simulink model "power_PSS_example2"  (R2022a)
settings: Solver=ode23tb  StartTime=0.0  StopTime=25  MaxStep=1/60  RelTol=1e-3  EnableMultiTasking=on
InitFcn:
  | paraset
values from neighbouring files (symbols this model uses):
  delta = 0.1    [paraset.m]
  k = 0.01    [paraset.m]
  kappa = 1    [paraset.m]
undefined symbols (not defined in the file or in its folder): D1, Delta
libraries: spsGenericPowerSystemStabilizerLib x8, spsLoadFlowBusLib x6, spsThreePhaseParallelRLCLoadLib x4, spsThreePhasePISectionLineLib x4, spsSynchronousMachinepuStandardLib x4, spsExcitationSystemLib x4, spsMultiBandPowerSystemStabilizerLib x4, spsSteamTurbineandGovernorLib x4, spsThreePhaseTransformerTwoWindingsLib x4, spsDistributedParametersLineLib x3, spsThreePhaseBreakerLib x2, spsThreePhaseVIMeasurementLib x2
(part 1 of 2)
settings Model: FPTRunName=Active  ExtModeTrigMode=oneshot  ExtModeArmWhenConnect=off  Creator=The MathWorks, Inc.  LastModifiedBy=matsu
settings SolverCC: AlgebraicLoopSolver=TrustRegion
settings DataIOCC: SaveFormat=Array  SaveOutput=off  SaveTime=off  ReturnWorkspaceOutputs=off  TimeSaveName=t  SignalLoggingName=sigsOut
settings OptimizationCC: BlockReduction=off  BooleanDataType=off  ExpressionDepthLimit=2147483647  InitFltsAndDblsToZero=on  LifeSpan=inf
settings DebuggingCC: UnderspecifiedInitializationDetection=Classic  MergeDetectMultiDrivingBlocksExec=none  SignalResolutionControl=TryResolveAllWithWarning  MultiTaskDSMMsg=warning  MultiTaskCondExecSysMsg=none  FcnCallInpInsideContextMsg=warning  UnconnectedInputMsg=warning  UnconnectedLineMsg=warning  StateNameClashWarn=warning  SFUnexpectedBacktrackingDiag=warning  SFNoUnconditionalDefaultTransitionDiag=warning  SFExecutionAtInitializationDiag=none  SFMachineParentedDataDiag=warning  ArithmeticOperatorsInVariantConditions=warning
settings HardwareCC: ProdBitPerPointer=32  ProdBitPerSizeT=32  ProdBitPerPtrDiffT=32  ProdLargestAtomicFloat=None  ProdIntDivRoundTo=Undefined  ProdEndianess=Unspecified  ProdWordSize=32  ProdHWDeviceType=32-bit Generic  TargetUnknown=on
settings ModelReferenceCC: PropagateSignalLabelsOutOfModel=off
settings SFSimCC: SimUseLocalCustomCode=off  CustomCodeUndefinedFunction=UseInterfaceOnly
settings RTWCC: RTWUseLocalCustomCode=off
settings CodeAppCC: StateflowObjectComments=on
settings GRTTargetCC: TargetLangStandard=C89/C90 (ANSI)  CombineOutputUpdateFcns=off  GRTInterface=on
settings ConfigComp: CovMetricSettings=dw  CovSaveCumulativeToWorkspaceVar=on  CovSaveSingleToWorkspaceVar=on  CovExternalEMLEnable=off  CovSFcnEnable=off
settings SimscapeCC: SimscapeNormalizeSystem=off

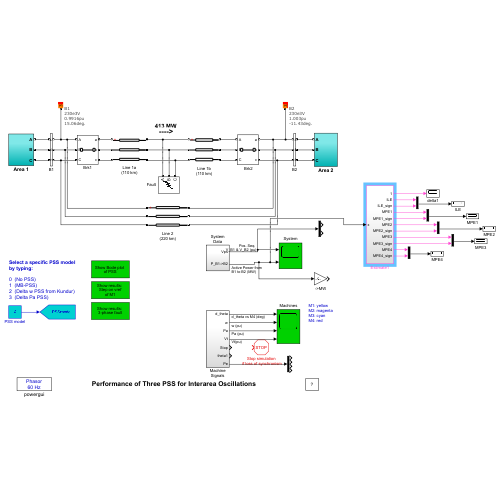
[thumbnail: Simulink's stored preview of the top-level diagram]
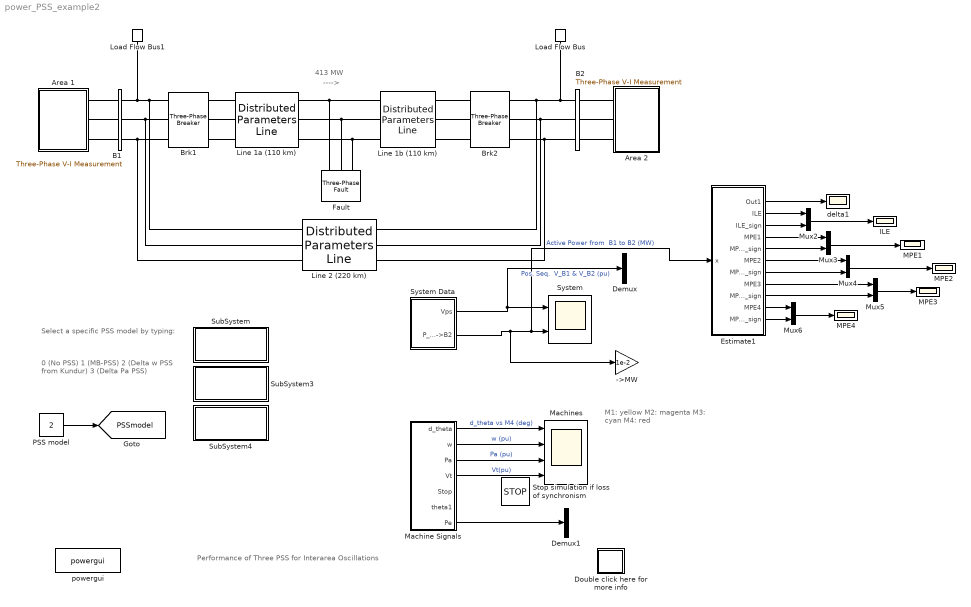
== system power_PSS_example2 ==
  note: Performance of Three PSS for Interarea Oscillations
  note: M1: yellow
      | M2: magenta
      | M3: cyan
      | M4: red
  note: ---->
  note: 413 MW
  note: Select a specific PSS model
      | by typing:
  note: 0  (No PSS)
      | 1  (MB-PSS)
      | 2  (Delta w PSS from Kundur)
      | 3  (Delta Pa PSS)
  " Brk2" : spsThreePhaseBreakerLib/Three-Phase Breaker  InitialState=closed  SwitchA=on  SwitchB=on  SwitchC=on  SwitchTimes=[1+6/60]  External=off  BreakerResistance=0.001  SnubberResistance=1e6  SnubberCapacitance=0  Measurements=None
      settings: AttributesFormatString=\n
  ->MW : Gain  Gain=1e-2  SaturateOnIntegerOverflow=on  OutDataTypeStr=Inherit: Same as input  ParamDataTypeStr=Inherit: Same as input
  Area 1 : Subsystem
  Area 2 : Subsystem
  B1 : spsThreePhaseVIMeasurementLib/Three-Phase V-I Measurement  VoltageMeasurement=phase-to-ground  SetLabelV=on  LabelV=Vabc_B1  Vpu=off  VpuLL=off  CurrentMeasurement=yes  SetLabelI=on  LabelI=Iabc_B1  Ipu=off  Pbase=100e6  Vbase=500e3  OutputType=Complex  PhasorSimulation=on  PSBequivalent=0
  B2 : spsThreePhaseVIMeasurementLib/Three-Phase V-I Measurement  VoltageMeasurement=phase-to-ground  SetLabelV=on  LabelV=Vabc_B2  Vpu=off  VpuLL=off  CurrentMeasurement=yes  SetLabelI=on  LabelI=Iabc_B2  Ipu=off  Pbase=100e6  Vbase=500e3  OutputType=Complex  PhasorSimulation=on  PSBequivalent=0
  Brk1 : spsThreePhaseBreakerLib/Three-Phase Breaker  InitialState=closed  SwitchA=on  SwitchB=on  SwitchC=on  SwitchTimes=[1+6/60]  External=off  BreakerResistance=0.001  SnubberResistance=inf  SnubberCapacitance=0  Measurements=None
      settings: AttributesFormatString=\n
  Demux : Demux  Outputs=2
  Demux1 : Demux
  Double click here for more info : Subsystem
      settings: OpenFcn=showdemo(bdroot(gcb))
      mask Display: disp('?')
  Estimate1 : Subsystem
  Fault : spsThreePhaseFaultLib/Three-Phase Fault  InitialStates=0  FaultA=on  FaultB=on  FaultC=on  GroundFault=on  SwitchTimes=[ 1 1+12/60]  External=off  SwitchStatus=NaN  FaultResistance=0.001  GroundResistance=0.001  SnubberResistance=inf  SnubberCapacitance=0  Measurements=None
  ILE : Scope
  Line 1a (110 km) : spsDistributedParametersLineLib/Distributed Parameters Line  Phases=3  Length=110  Frequency=60  Resistance=[0.0001*529 1.61]  Inductance=[0.001*529/(377) 0.0061]  Capacitance=[0.00175/529/(377) 5.2489e-9]  x1=[2.32637796386765e-08 228065.253428989 228064.749078735;376.991118430775 376.991118430775 376.991118430775;-1.32137751305166 0.640983254504953 -0.929809730908466]  x2=[1.11620897117682e-08 225636.373835133 225635.928060063;376.991118430775 376.991118430775 376.991118430775;-2.82766360003001 0.407410565435935 -1.16338269104508]  x3=[5.86477000241848e-11 336.016991920685 336.017366292842;376.991118430775 376.991118430775 376.991118430775;1.18739859871112 -2.54715832281008 2.16523641414879]  x4=[7.98351229776034e-11 1450.97195175507 1450.96987265642;376.991118430775 376.991118430775 376.991118430775;-1.93500873855342 0.484728016775275 -1.08606444535416]  x5=0.000622431770558027  V1=ones(3,3)  V2=ones(3,3)  I1=ones(3,3)  I2=ones(3,3)  nHarmo=1  Measurements=None  Decoupling=off  VsMag0=0  VrMag0=0  VsAngle0=0  VrAngle0=0  IsMag0=0  IrMag0=0  IsAngle0=0  IrAngle0=0
      settings: AttributesFormatString=\n  SourceProductBaseCode=PS
  Line 1b (110 km) : spsDistributedParametersLineLib/Distributed Parameters Line  Phases=3  Length=110  Frequency=60  Resistance=[0.0001*529 1.61]  Inductance=[0.001*529/(377) 0.0061]  Capacitance=[0.00175/529/(377) 5.2489e-9]  x1=[1.11620897117682e-08 225636.373835133 225635.928060063;376.991118430775 376.991118430775 376.991118430775;-2.82766360003001 0.407410565435935 -1.16338269104508]  x2=[3.02591716623452e-08 230641.661959582 230641.282002309;376.991118430775 376.991118430775 376.991118430775;2.60366923923542 0.178614649234263 -1.39217874313558]  x3=[7.01764132995704e-11 348.868575534709 348.868934214032;376.991118430775 376.991118430775 376.991118430775;1.39792395828996 -2.40713389014301 2.30526080396357]  x4=[6.82690946295777e-11 1438.06126547657 1438.05920047338;376.991118430775 376.991118430775 376.991118430775;-2.20731822356487 0.338658780991479 -1.23213368558469]  x5=0.000622431770558027  V1=ones(3,3)  V2=ones(3,3)  I1=ones(3,3)  I2=ones(3,3)  nHarmo=1  Measurements=None  Decoupling=off  VsMag0=0  VrMag0=0  VsAngle0=0  VrAngle0=0  IsMag0=0  IrMag0=0  IsAngle0=0  IrAngle0=0
      settings: AttributesFormatString=\n  SourceProductBaseCode=PS
  Line 2 (220 km) : spsDistributedParametersLineLib/Distributed Parameters Line  Phases=3  Length=220  Frequency=60  Resistance=[0.0001*529 1.61]  Inductance=[0.001*529/(377) 0.0061]  Capacitance=[0.00175/529/(377) 5.2489e-9]  x1=[1.24832194921319e-08 228066.159790877 228065.655439803;376.991118430775 376.991118430775 376.991118430775;-1.93381850732894 0.495470291490433 -1.0753226939196]  x2=[2.89327326949073e-08 230640.806586718 230640.426630747;376.991118430775 376.991118430775 376.991118430775;-1.98298217607113 0.0331007543902468 -1.53769263798565]  x3=[3.07384841100258e-11 335.618352779838 335.618719794473;376.991118430775 376.991118430775 376.991118430775;-2.78833319776652 -2.69313965469147 2.01925506825551]  x4=[1.71224684396664e-11 1425.65369023884 1425.6516439244;376.991118430775 376.991118430775 376.991118430775;-0.949321440854882 0.193205204918508 -1.37758726043151]  x5=0.00124486354111605  V1=ones(3,3)  V2=ones(3,3)  I1=ones(3,3)  I2=ones(3,3)  nHarmo=1  Measurements=None  Decoupling=off  VsMag0=0  VrMag0=0  VsAngle0=0  VrAngle0=0  IsMag0=0  IrMag0=0  IsAngle0=0  IrAngle0=0
      settings: AttributesFormatString=\n  SourceProductBaseCode=PS
  Load Flow Bus : spsLoadFlowBusLib/Load Flow Bus  LConnTagsString=a  Phases=single  Connectors=on one side  ID=B2  Vbase=230e3  Vref=1  Vangle=0  VLF=1.003  VLFb=1  VLFc=1  angleLF=-11.43  angleLFb=0  angleLFc=0
      settings: AttributesFormatString=%<ID>\n%<Vbase>V\n%<VLF>pu\n%<angleLF>deg.  SourceProductBaseCode=PS
  Load Flow Bus1 : spsLoadFlowBusLib/Load Flow Bus  LConnTagsString=a  Phases=single  Connectors=on one side  ID=B1  Vbase=230e3  Vref=1  Vangle=0  VLF=0.9916  VLFb=1  VLFc=1  angleLF=15.06  angleLFb=0  angleLFc=0
      settings: AttributesFormatString=%<ID>\n%<Vbase>V\n%<VLF>pu\n%<angleLF>deg.  SourceProductBaseCode=PS
  MPE{1..4} (4 alike) : Scope
  Machine Signals : Subsystem
  Machines : Scope  NumInputPorts=4
  Mux{2..6} (5 alike) : Mux  Inputs=2
  PSS model : Constant  Value=2
  Stop simulation if loss of synchronism : Stop
  SubSystem : Subsystem
      settings: OpenFcn=openfig('psbPSSbode.fig');
      mask Display: disp('Show Bode plot \nof PSS')
  SubSystem3 : Subsystem
      settings: OpenFcn=openfig('psbPSSstep.fig');
      mask Display: disp('Show results: \nStep on vref\nof M1')
  SubSystem4 : Subsystem
      settings: OpenFcn=openfig('psbPSSfault.fig');
      mask Display: disp('Show results: \n3-phase fault')
  System : Scope  NumInputPorts=2
  System Data : Subsystem
  delta1 : Scope
  powergui : spspowerguiLib/powergui  Priority=2  SimulationMode=Phasor  SampleTime=0  frequency=60  Iterations=50  frequencyindice=60  Pbase=100e6  ErrMax=0.0001  UnitsV=kV  UnitsW=MW  buscounter=0  FunctionMessages=off  echomessages=off  EnableUseOfTLC=off  CurrentSourceSwitches=off  DisableSnubberDevices=off  DisableRonSwitches=off  DisableVfSwitches=off  DisplayEquations=off  AutomaticDiscreteSolvers=off  SolverType=Tustin  Interpol=off  ExternalGateDelay=off  methode=off  Ts=0  x0status=blocks  SPID=off  SwTol=0  HookPort=off  NonlinearTolerance=1e-4  nMaxIteration=100  ContinueOnMaxIteration=off  RestoreLinks=warning  ResistiveCurrentMeasurement=off  Frange=logspace(0,3,50)  Ylog=off  Xlog=off  ShowGrid=off  save=off  variable=ZData  structure=0  ZoomFFT=on  StartTime=0.0  cycles=1  DisplayStyle=1  fundamental=60  FreqAxis=off  MaxFrequency=1000  frequencyindicesteady=1  RmsSteady=1  display=off
  tag scope: PSSmodel=global
  wires:
  Machine Signals/1(d_theta) -> Machines/1  "d_theta vs M4 (deg)"
  Machine Signals/2(w) -> Machines/2  "w (pu)"
  Machine Signals/3(Pa) -> Machines/3  "Pa (pu)"
  Machine Signals/4(Vt) -> Machines/4  "Vt(pu)"
  System Data/1(Vps) -> Demux/1, System/1  "Pos. Seq.  V_B1 & V_B2 (pu)"
  System Data/2(P_B1->B2) -> ->MW/1, Estimate1/1(x), System/2  "Active Power from  B1 to B2 (MW)"
  PSS model/1 -> [PSSmodel]
  Estimate1/4(MPE1) -> Mux3/1
  Estimate1/5(MPE1_sign) -> Mux3/2
  Estimate1/2(ILE) -> Mux2/1
  Mux2/1 -> ILE/1
  Mux5/1 -> MPE3/1
  Estimate1/9(MPE3_sign) -> Mux5/2
  Estimate1/8(MPE3) -> Mux5/1
  Mux6/1 -> MPE4/1
  Estimate1/11(MPE4_sign) -> Mux6/2
  Estimate1/7(MPE2_sign) -> Mux4/2
  Estimate1/1(Out1) -> delta1/1
  Estimate1/3(ILE_sign) -> Mux2/2
  Estimate1/6(MPE2) -> Mux4/1
  Mux4/1 -> MPE2/1
  Estimate1/10(MPE4) -> Mux6/1
  Mux3/1 -> MPE1/1
  Machine Signals/7(Pe) -> Demux1/1
  connections:
  Brk1/RConn1 -- Line 1a (110 km)/LConn1
  Brk1/RConn2 -- Line 1a (110 km)/LConn2
  Brk1/RConn3 -- Line 1a (110 km)/LConn3
  Line 1b (110 km)/LConn1 -- Line 1a (110 km)/RConn1 -- Fault/LConn1
  Line 1b (110 km)/LConn2 -- Line 1a (110 km)/RConn2 -- Fault/LConn2
  Line 1a (110 km)/RConn3 -- Line 1b (110 km)/LConn3 -- Fault/LConn3
  Line 1b (110 km)/RConn1 -- " Brk2"/LConn1
  Line 1b (110 km)/RConn2 -- " Brk2"/LConn2
  Line 1b (110 km)/RConn3 -- " Brk2"/LConn3
  Area 1/RConn2 -- B1/LConn2
  Area 1/RConn1 -- B1/LConn1
  Area 1/RConn3 -- B1/LConn3
  B1/RConn2 -- Brk1/LConn2 -- Line 2 (220 km)/LConn2
  B1/RConn1 -- Brk1/LConn1 -- Line 2 (220 km)/LConn1 -- Load Flow Bus1/LConn1
  B1/RConn3 -- Brk1/LConn3 -- Line 2 (220 km)/LConn3
  B2/RConn2 -- Area 2/LConn2
  B2/RConn1 -- Area 2/LConn1
  B2/RConn3 -- Area 2/LConn3
  B2/LConn2 -- " Brk2"/RConn2 -- Line 2 (220 km)/RConn2
  B2/LConn1 -- " Brk2"/RConn1 -- Line 2 (220 km)/RConn1 -- Load Flow Bus/LConn1
  B2/LConn3 -- " Brk2"/RConn3 -- Line 2 (220 km)/RConn3

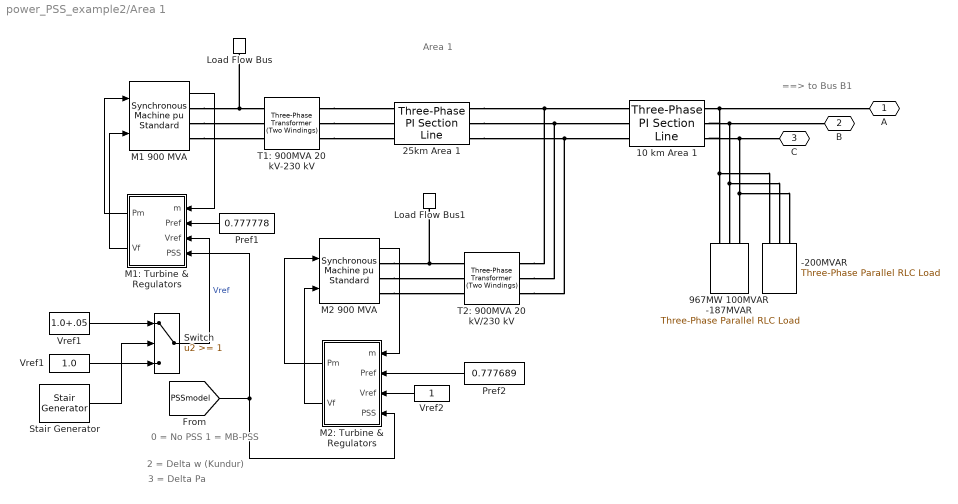
== system power_PSS_example2/Area 1 ==
  note: Area 1
  note: ==> to Bus B1
  note: 0 = No PSS
      | 1 = MB-PSS
  note: 3 = Delta Pa
  note: 2 = Delta w (Kundur)
  -200MVAR : spsThreePhaseParallelRLCLoadLib/Three-Phase Parallel RLC Load  LConnTagsString=A|B|C  Configuration=Y (grounded)  NominalVoltage=230e3  Vabc=[1e3 1e3 1e3]  Vabcp=[1e3 1e3 1e3]  NominalFrequency=60  UnbalancedPower=off  ActivePower=0  InductivePower=0  CapacitivePower=200e6  Pabc=[10e3 9e3 11e3]  QLabc=[100 90 110]  QCabc=[100 90 110]  Pabcp=[10e3 9e3 11e3]  QLabcp=[100 90 110]  QCabcp=[100 90 110]  Measurements=None  LoadType=constant Z
  10 km Area 1 : spsThreePhasePISectionLineLib/Three-Phase PI Section Line  LConnTagsString=a|b|c  RConnTagsString=A|B|C  Length=10  Frequency=60  Resistances=[0.0001*529 1.61]  Inductances=[0.001*529/(377) 0.0061]  Capacitances=[0.00175/529/(377) 5.2489e-9]
  25km Area 1 : spsThreePhasePISectionLineLib/Three-Phase PI Section Line  LConnTagsString=a|b|c  RConnTagsString=A|B|C  Length=25  Frequency=60  Resistances=[0.0001*529 1.61]  Inductances=[0.001*529/(377) 0.0061]  Capacitances=[0.00175/529/(377) 5.2489e-9]
  967MW 100MVAR -187MVAR : spsThreePhaseParallelRLCLoadLib/Three-Phase Parallel RLC Load  LConnTagsString=A|B|C  Configuration=Y (grounded)  NominalVoltage=230e3  Vabc=[1e3 1e3 1e3]  Vabcp=[1e3 1e3 1e3]  NominalFrequency=60  UnbalancedPower=off  ActivePower=967000000  InductivePower=100e6  CapacitivePower=187e6  Pabc=[10e3 9e3 11e3]  QLabc=[100 90 110]  QCabc=[100 90 110]  Pabcp=[10e3 9e3 11e3]  QLabcp=[100 90 110]  QCabcp=[100 90 110]  Measurements=None  LoadType=constant Z
  Load Flow Bus : spsLoadFlowBusLib/Load Flow Bus  LConnTagsString=a  Phases=single  Connectors=on one side  ID=M1_Area1  Vbase=20e3  Vref=1  Vangle=0  VLF=1  VLFb=1  VLFc=1  angleLF=10.22  angleLFb=0  angleLFc=0
      settings: AttributesFormatString=%<ID>\n%<Vbase>V\n%<VLF>pu\n%<angleLF>deg.  SourceProductBaseCode=PS
  Load Flow Bus1 : spsLoadFlowBusLib/Load Flow Bus  LConnTagsString=a  Phases=single  Connectors=on one side  ID=M2_Area1  Vbase=20e3  Vref=1  Vangle=0  VLF=1  VLFb=1  VLFc=1  angleLF=0  angleLFb=0  angleLFc=0
      settings: AttributesFormatString=%<ID>\n%<Vbase>V\n%<VLF>pu\n%<angleLF>deg.  SourceProductBaseCode=PS
  M1 900 MVA : spsSynchronousMachinepuStandardLib/Synchronous Machine pu Standard  PresetModel=No  MechanicalLoad=Mechanical power Pm  ShowDetailedParameters=on  RotorType=Round  Units=per unit standard parameters  MeasurementBus=off  NominalParameters="[900E6  20000   60 ]"  Reactances1=[1.8 .3 .25 1.7 .55 .25 .2]  Reactances2=[ 1.305, 0.296, 0.252, 0.474, 0.243, 0.18 ]  dAxisTimeConstants=Open-circuit  qAxisTimeConstants=Open-circuit  TimeConstants1=[]  TimeConstants2=[8 .03 .4 .05]  TimeConstants3=[]  TimeConstants4=[]  TimeConstants5=[ 1.01, 0.053, 0.1 ]  TimeConstants6=[]  TimeConstants7=[]  TimeConstants8=[]  StatorResistance=0.0025  Mechanical=[ 6.5 0 4]  PolePairs=4  InitialConditions=[0 -31.4247 0.784453 0.784453 0.784453 2.7401 -117.26 122.74 1.83395]  SetSaturation=off  Saturation=[0.6404,0.7127,0.8441,0.9214,0.9956,1.082,1.19,1.316,1.457;0.7,0.7698,0.8872,0.9466,0.9969,1.046,1.1,1.151,1.201]  LoadFlowParameters=[1 700000000 0 0 0]  TsPowergui=0  TsBlock=-1  IterativeModel=Trapezoidal non iterative  IterativeDiscreteModel=Trapezoidal non iterative  BusType=PV  Pref=700000000  Qref=0  Qmin=-Inf  Qmax=Inf  PLF=0  QLF=0
      settings: SourceProductBaseCode=PS
  M1: Turbine & Regulators : Subsystem
  M2 900 MVA : spsSynchronousMachinepuStandardLib/Synchronous Machine pu Standard  PresetModel=No  MechanicalLoad=Mechanical power Pm  ShowDetailedParameters=on  RotorType=Round  Units=per unit standard parameters  MeasurementBus=off  NominalParameters="[900E6  20000   60 ]"  Reactances1=[1.8 .3 .25 1.7 .55 .25 .2]  Reactances2=[ 1.305, 0.296, 0.252, 0.474, 0.243, 0.18 ]  dAxisTimeConstants=Open-circuit  qAxisTimeConstants=Open-circuit  TimeConstants1=[]  TimeConstants2=[8 .03 .4 .05]  TimeConstants3=[]  TimeConstants4=[]  TimeConstants5=[ 1.01, 0.053, 0.1 ]  TimeConstants6=[]  TimeConstants7=[]  TimeConstants8=[]  StatorResistance=0.0025  Mechanical=[ 6.5 0 4]  PolePairs=4  InitialConditions=[0 -42.8075 0.788608 0.788608 0.788608 -9.54571 -129.546 110.454 1.86756]  SetSaturation=off  Saturation=[0.6404,0.7127,0.8441,0.9214,0.9956,1.082,1.19,1.316,1.457;0.7,0.7698,0.8872,0.9466,0.9969,1.046,1.1,1.151,1.201]  LoadFlowParameters=[2 700000000 0 0 0]  TsPowergui=0  TsBlock=-1  IterativeModel=Trapezoidal non iterative  IterativeDiscreteModel=Trapezoidal non iterative  BusType=swing  Pref=0  Qref=0  Qmin=-Inf  Qmax=Inf  PLF=0  QLF=0
      settings: SourceProductBaseCode=PS
  M2: Turbine & Regulators : Subsystem
  Pref1 : Constant  Value=0.777778
  Pref2 : Constant  Value=0.777689
  Stair Generator : spsStairGeneratorLib/Stair Generator  t=[0 1 1.2]*100  e=[0 1 0 ]  Ts=0
  Switch : Switch  Threshold=1  SaturateOnIntegerOverflow=off
  T1: 900MVA 20 kV-230 kV : spsThreePhaseTransformerTwoWindingsLib/Three-Phase Transformer (Two Windings)  Winding1Connection=Delta (D1)  Winding2Connection=Yg  CoreType=Three single-phase transformers  SetSaturation=off  Hysteresis=off  DataFile='hysteresis'  SetInitialFlux=off  Measurements=None  UNITS=pu  NominalPower="[ 900e6   60 ]"  Winding1="[ 20e3  1e-6   0  ]"  Winding2="[ 230e3  1e-6   0.15 ]"  Rm=500  Lm=500  L0=0.5  Saturation="[ 0,0  ;  0.005,1.2  ;  1.0,1.4 ]"  InitialFluxes=[ 0.8 , -0.8 , 0.7 ]  BreakLoop=off  DiscreteSolver=Trapezoidal iterative  DataType=off  TransfoNumber=0
  T2: 900MVA 20 kV/230 kV : spsThreePhaseTransformerTwoWindingsLib/Three-Phase Transformer (Two Windings)  Winding1Connection=Delta (D1)  Winding2Connection=Yg  CoreType=Three single-phase transformers  SetSaturation=off  Hysteresis=off  DataFile='hysteresis'  SetInitialFlux=off  Measurements=None  UNITS=pu  NominalPower=[ 900e6 60 ]  Winding1="[ 20e3 1e-6  0.0]"  Winding2=[ 230e3 1e-6 0.15]  Rm=500  Lm=500  L0=0.5  Saturation="[ 0,0  ;  0.005,1.2  ;  1.0,1.4 ]"  InitialFluxes=[ 0.8 , -0.8 , 0.7 ]  BreakLoop=off  DiscreteSolver=Trapezoidal iterative  DataType=off  TransfoNumber=0
  Vref1 : Constant  Value=1.0
  "Vref1 " : Constant  Value=1.0+.05
  Vref2 : Constant
  " A" : PMIOPort  Side=Right
  " B" : PMIOPort  Port=2  Side=Right
  " C" : PMIOPort  Port=3  Side=Right
  wires:
  Pref1/1 -> M1: Turbine & Regulators/2(Pref)
  Switch/1 -> M1: Turbine & Regulators/3(Vref)  "Vref"
  Stair Generator/1 -> Switch/2
  [PSSmodel] -> M1: Turbine & Regulators/4(PSS), M2: Turbine & Regulators/4(PSS)
  Pref2/1 -> M2: Turbine & Regulators/2(Pref)
  Vref2/1 -> M2: Turbine & Regulators/3(Vref)
  Vref1/1 -> Switch/3
  "Vref1 "/1 -> Switch/1
  M2 900 MVA/1 -> M2: Turbine & Regulators/1(m)
  M2: Turbine & Regulators/1(Pm) -> M2 900 MVA/1
  M2: Turbine & Regulators/2(Vf) -> M2 900 MVA/2
  M1: Turbine & Regulators/1(Pm) -> M1 900 MVA/1
  M1: Turbine & Regulators/2(Vf) -> M1 900 MVA/2
  M1 900 MVA/1 -> M1: Turbine & Regulators/1(m)
  connections:
  T1: 900MVA 20 kV-230 kV/RConn1 -- 25km Area 1/LConn1
  T1: 900MVA 20 kV-230 kV/RConn2 -- 25km Area 1/LConn2
  M2 900 MVA/RConn1 -- T2: 900MVA 20 kV/230 kV/LConn1 -- Load Flow Bus1/LConn1
  M2 900 MVA/RConn2 -- T2: 900MVA 20 kV/230 kV/LConn2
  M2 900 MVA/RConn3 -- T2: 900MVA 20 kV/230 kV/LConn3
  T1: 900MVA 20 kV-230 kV/RConn3 -- 25km Area 1/LConn3
  10 km Area 1/RConn1 -- " A"/RConn1 -- 967MW 100MVAR -187MVAR/LConn1 -- -200MVAR/LConn1
  10 km Area 1/RConn2 -- " B"/RConn1 -- 967MW 100MVAR -187MVAR/LConn2 -- -200MVAR/LConn2
  10 km Area 1/RConn3 -- " C"/RConn1 -- 967MW 100MVAR -187MVAR/LConn3 -- -200MVAR/LConn3
  M1 900 MVA/RConn1 -- T1: 900MVA 20 kV-230 kV/LConn1 -- Load Flow Bus/LConn1
  M1 900 MVA/RConn2 -- T1: 900MVA 20 kV-230 kV/LConn2
  M1 900 MVA/RConn3 -- T1: 900MVA 20 kV-230 kV/LConn3
  25km Area 1/RConn2 -- 10 km Area 1/LConn2 -- T2: 900MVA 20 kV/230 kV/RConn2
  25km Area 1/RConn1 -- 10 km Area 1/LConn1 -- T2: 900MVA 20 kV/230 kV/RConn1
  25km Area 1/RConn3 -- 10 km Area 1/LConn3 -- T2: 900MVA 20 kV/230 kV/RConn3

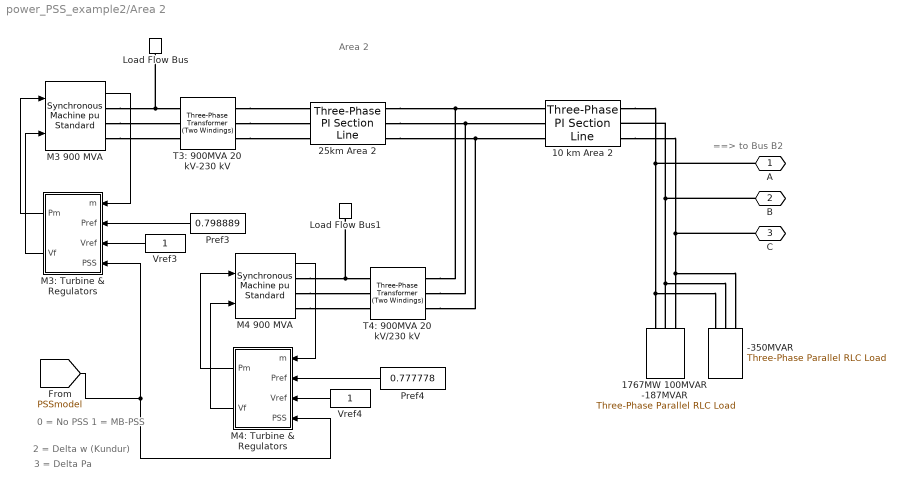
== system power_PSS_example2/Area 2 ==
  note: 2 = Delta w (Kundur)
  note: 3 = Delta Pa
  note: 0 = No PSS
      | 1 = MB-PSS
  note: ==> to Bus B2
  note: Area 2
  -350MVAR : spsThreePhaseParallelRLCLoadLib/Three-Phase Parallel RLC Load  LConnTagsString=A|B|C  Configuration=Y (grounded)  NominalVoltage=230e3  Vabc=[1e3 1e3 1e3]  Vabcp=[1e3 1e3 1e3]  NominalFrequency=60  UnbalancedPower=off  ActivePower=0  InductivePower=0  CapacitivePower=350e6  Pabc=[10e3 9e3 11e3]  QLabc=[100 90 110]  QCabc=[100 90 110]  Pabcp=[10e3 9e3 11e3]  QLabcp=[100 90 110]  QCabcp=[100 90 110]  Measurements=None  LoadType=constant Z
  10 km Area 2 : spsThreePhasePISectionLineLib/Three-Phase PI Section Line  LConnTagsString=a|b|c  RConnTagsString=A|B|C  Length=10  Frequency=60  Resistances=[0.0001*529 1.61]  Inductances=[0.001*529/(377) 0.0061]  Capacitances=[0.00175/529/(377) 5.2489e-9]
  1767MW 100MVAR -187MVAR : spsThreePhaseParallelRLCLoadLib/Three-Phase Parallel RLC Load  LConnTagsString=A|B|C  Configuration=Y (grounded)  NominalVoltage=230e3  Vabc=[1e3 1e3 1e3]  Vabcp=[1e3 1e3 1e3]  NominalFrequency=60  UnbalancedPower=off  ActivePower=1767000000  InductivePower=100e6  CapacitivePower=187e6  Pabc=[10e3 9e3 11e3]  QLabc=[100 90 110]  QCabc=[100 90 110]  Pabcp=[10e3 9e3 11e3]  QLabcp=[100 90 110]  QCabcp=[100 90 110]  Measurements=None  LoadType=constant Z
  25km Area 2 : spsThreePhasePISectionLineLib/Three-Phase PI Section Line  LConnTagsString=a|b|c  RConnTagsString=A|B|C  Length=25  Frequency=60  Resistances=[0.0001*529 1.61]  Inductances=[0.001*529/(377) 0.0061]  Capacitances=[0.00175/529/(377) 5.2489e-9]
  Load Flow Bus : spsLoadFlowBusLib/Load Flow Bus  LConnTagsString=a  Phases=single  Connectors=on one side  ID=M3_Area2  Vbase=20e3  Vref=1  Vangle=0  VLF=1  VLFb=1  VLFc=1  angleLF=-15.88  angleLFb=0  angleLFc=0
      settings: AttributesFormatString=%<ID>\n%<Vbase>V\n%<VLF>pu\n%<angleLF>deg.  SourceProductBaseCode=PS
  Load Flow Bus1 : spsLoadFlowBusLib/Load Flow Bus  LConnTagsString=a  Phases=single  Connectors=on one side  ID=M4_Area2  Vbase=20e3  Vref=1  Vangle=0  VLF=1  VLFb=1  VLFc=1  angleLF=-26.53  angleLFb=0  angleLFc=0
      settings: AttributesFormatString=%<ID>\n%<Vbase>V\n%<VLF>pu\n%<angleLF>deg.  SourceProductBaseCode=PS
  M3 900 MVA : spsSynchronousMachinepuStandardLib/Synchronous Machine pu Standard  PresetModel=No  MechanicalLoad=Mechanical power Pm  ShowDetailedParameters=on  RotorType=Round  Units=per unit standard parameters  MeasurementBus=off  NominalParameters="[900E6  20000   60 ]"  Reactances1=[1.8 .3 .25 1.7 .55 .25 .2]  Reactances2=[ 1.305, 0.296, 0.252, 0.474, 0.243, 0.18 ]  dAxisTimeConstants=Open-circuit  qAxisTimeConstants=Open-circuit  TimeConstants1=[]  TimeConstants2=[8 .03 .4 .05]  TimeConstants3=[]  TimeConstants4=[]  TimeConstants5=[ 1.01, 0.053, 0.1 ]  TimeConstants6=[]  TimeConstants7=[]  TimeConstants8=[]  StatorResistance=0.0025  Mechanical=[ 6.175 0 4]  PolePairs=4  InitialConditions=[0 -56.3243 0.8041 0.8041 0.8041 -22.4087 -142.409 97.5913 1.85092]  SetSaturation=off  Saturation=[0.6404,0.7127,0.8441,0.9214,0.9956,1.082,1.19,1.316,1.457;0.7,0.7698,0.8872,0.9466,0.9969,1.046,1.1,1.151,1.201]  LoadFlowParameters=[1 719000000 0 0 0]  TsPowergui=0  TsBlock=-1  IterativeModel=Trapezoidal non iterative  IterativeDiscreteModel=Trapezoidal non iterative  BusType=PV  Pref=719000000  Qref=0  Qmin=-Inf  Qmax=Inf  PLF=0  QLF=0
      settings: SourceProductBaseCode=PS
  M3: Turbine & Regulators : Subsystem
  M4 900 MVA : spsSynchronousMachinepuStandardLib/Synchronous Machine pu Standard  PresetModel=No  MechanicalLoad=Mechanical power Pm  ShowDetailedParameters=on  RotorType=Round  Units=per unit standard parameters  MeasurementBus=off  NominalParameters="[900E6  20000   60 ]"  Reactances1=[1.8 .3 .25 1.7 .55 .25 .2]  Reactances2=[ 1.305, 0.296, 0.252, 0.474, 0.243, 0.18 ]  dAxisTimeConstants=Open-circuit  qAxisTimeConstants=Open-circuit  TimeConstants1=[]  TimeConstants2=[8 .03 .4 .05]  TimeConstants3=[]  TimeConstants4=[]  TimeConstants5=[ 1.01, 0.053, 0.1 ]  TimeConstants6=[]  TimeConstants7=[]  TimeConstants8=[]  StatorResistance=0.0025  Mechanical=[ 6.175 0 4]  PolePairs=4  InitialConditions=[0 -67.7513 0.783185 0.783185 0.783185 -33.268 -153.268 86.732 1.82209]  SetSaturation=off  Saturation=[0.6404,0.7127,0.8441,0.9214,0.9956,1.082,1.19,1.316,1.457;0.7,0.7698,0.8872,0.9466,0.9969,1.046,1.1,1.151,1.201]  LoadFlowParameters=[1 700000000 0 0 0]  TsPowergui=0  TsBlock=-1  IterativeModel=Trapezoidal non iterative  IterativeDiscreteModel=Trapezoidal non iterative  BusType=PV  Pref=700000000  Qref=0  Qmin=-Inf  Qmax=Inf  PLF=0  QLF=0
      settings: SourceProductBaseCode=PS
  M4: Turbine & Regulators : Subsystem
  Pref3 : Constant  Value=0.798889
  Pref4 : Constant  Value=0.777778
  T3: 900MVA 20 kV-230 kV : spsThreePhaseTransformerTwoWindingsLib/Three-Phase Transformer (Two Windings)  Winding1Connection=Delta (D1)  Winding2Connection=Yg  CoreType=Three single-phase transformers  SetSaturation=off  Hysteresis=off  DataFile='hysteresis'  SetInitialFlux=off  Measurements=None  UNITS=pu  NominalPower="[ 900e6   60 ]"  Winding1="[ 20e3  1e-6   0  ]"  Winding2="[ 230e3  1e-6   0.15 ]"  Rm=500  Lm=500  L0=0.5  Saturation="[ 0,0  ;  0.005,1.2  ;  1.0,1.4 ]"  InitialFluxes=[ 0.8 , -0.8 , 0.7 ]  BreakLoop=off  DiscreteSolver=Trapezoidal iterative  DataType=off  TransfoNumber=0
  T4: 900MVA 20 kV/230 kV : spsThreePhaseTransformerTwoWindingsLib/Three-Phase Transformer (Two Windings)  Winding1Connection=Delta (D1)  Winding2Connection=Yg  CoreType=Three single-phase transformers  SetSaturation=off  Hysteresis=off  DataFile='hysteresis'  SetInitialFlux=off  Measurements=None  UNITS=pu  NominalPower=[ 900e6 60 ]  Winding1="[ 20e3 1e-6  0.0]"  Winding2=[ 230e3 1e-6 0.15]  Rm=500  Lm=500  L0=0.5  Saturation="[ 0,0  ;  0.005,1.2  ;  1.0,1.4 ]"  InitialFluxes=[ 0.8 , -0.8 , 0.7 ]  BreakLoop=off  DiscreteSolver=Trapezoidal iterative  DataType=off  TransfoNumber=0
  Vref3 : Constant
  Vref4 : Constant
  A : PMIOPort  Side=Left
  B : PMIOPort  Port=2  Side=Left
  C : PMIOPort  Port=3  Side=Left
  wires:
  [PSSmodel] -> M3: Turbine & Regulators/4(PSS), M4: Turbine & Regulators/4(PSS)
  Pref3/1 -> M3: Turbine & Regulators/2(Pref)
  Vref3/1 -> M3: Turbine & Regulators/3(Vref)
  Pref4/1 -> M4: Turbine & Regulators/2(Pref)
  Vref4/1 -> M4: Turbine & Regulators/3(Vref)
  M3 900 MVA/1 -> M3: Turbine & Regulators/1(m)
  M3: Turbine & Regulators/2(Vf) -> M3 900 MVA/2
  M3: Turbine & Regulators/1(Pm) -> M3 900 MVA/1
  M4: Turbine & Regulators/1(Pm) -> M4 900 MVA/1
  M4: Turbine & Regulators/2(Vf) -> M4 900 MVA/2
  M4 900 MVA/1 -> M4: Turbine & Regulators/1(m)
  connections:
  M3 900 MVA/RConn3 -- T3: 900MVA 20 kV-230 kV/LConn3
  M3 900 MVA/RConn2 -- T3: 900MVA 20 kV-230 kV/LConn2
  M3 900 MVA/RConn1 -- T3: 900MVA 20 kV-230 kV/LConn1 -- Load Flow Bus/LConn1
  T3: 900MVA 20 kV-230 kV/RConn3 -- 25km Area 2/LConn3
  M4 900 MVA/RConn3 -- T4: 900MVA 20 kV/230 kV/LConn3
  M4 900 MVA/RConn2 -- T4: 900MVA 20 kV/230 kV/LConn2
  M4 900 MVA/RConn1 -- T4: 900MVA 20 kV/230 kV/LConn1 -- Load Flow Bus1/LConn1
  T3: 900MVA 20 kV-230 kV/RConn2 -- 25km Area 2/LConn2
  T3: 900MVA 20 kV-230 kV/RConn1 -- 25km Area 2/LConn1
  25km Area 2/RConn2 -- 10 km Area 2/LConn2 -- T4: 900MVA 20 kV/230 kV/RConn2
  25km Area 2/RConn1 -- 10 km Area 2/LConn1 -- T4: 900MVA 20 kV/230 kV/RConn1
  25km Area 2/RConn3 -- 10 km Area 2/LConn3 -- T4: 900MVA 20 kV/230 kV/RConn3
  10 km Area 2/RConn1 -- 1767MW 100MVAR -187MVAR/LConn1 -- -350MVAR/LConn1 -- A/RConn1
  1767MW 100MVAR -187MVAR/LConn2 -- -350MVAR/LConn2 -- 10 km Area 2/RConn2 -- B/RConn1
  10 km Area 2/RConn3 -- 1767MW 100MVAR -187MVAR/LConn3 -- -350MVAR/LConn3 -- C/RConn1

== system power_PSS_example2/Double click here for more info ==

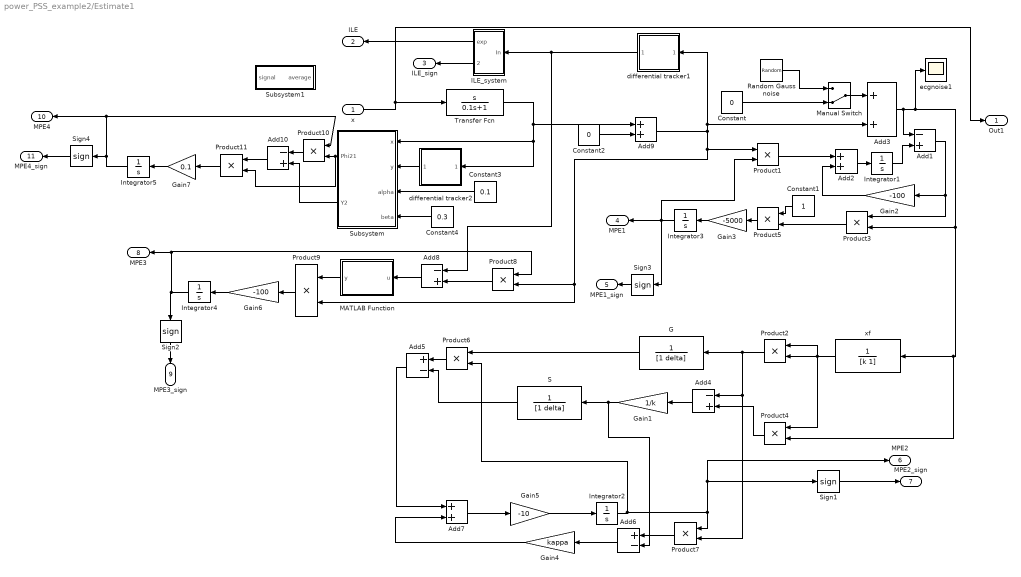
== system power_PSS_example2/Estimate1 ==
  x : Inport
  Add{1,4,8,10} (4 alike) : Sum  Inputs=-+
  Add{2..3,7,9} (4 alike) : Sum
  Add5 : Sum  Inputs=+-
  Add6 : Sum  Inputs=+-
  Constant : Constant  Value=0
  Constant1 : Constant
  Constant2 : Constant  Value=0
  Constant3 : Constant  Value=0.1
  Constant4 : Constant  Value=0.3
  G : TransferFcn  Denominator=[1 delta]
  Gain1 : Gain  Gain=1/k
  Gain2 : Gain  Gain=-100
  Gain3 : Gain  Gain=-5000
  Gain4 : Gain  Gain=kappa
  Gain5 : Gain  Gain=-10
  Gain6 : Gain  Gain=-100
  Gain7 : Gain  Gain=0.1
  ILE_system : Subsystem
  Integrator{1..5} (5 alike) : Integrator
  MATLAB Function : MATLAB Function  TreatAsAtomicUnit=on
  Manual Switch : ManualSwitch  CurrentSetting=0
  Product{1..11} (11 alike) : Product  RndMeth=Zero
  Random Gauss noise : RandomNumber  Variance=0.0001  SampleTime=0
  S : TransferFcn  Denominator=[1 delta]
  Sign{1..4} (4 alike) : Signum
  Subsystem : Subsystem
  Subsystem1 : Subsystem
  Transfer Fcn : TransferFcn  Numerator=[1 0]  Denominator=[0.1 1]
  differential tracker1 : Subsystem
  differential tracker2 : Subsystem
  ecgnoise1 : Scope
  xf : TransferFcn  Denominator=[k 1]
  Out1 : Outport  VectorParamsAs1DForOutWhenUnconnected=off
  ILE : Outport  Port=2  VectorParamsAs1DForOutWhenUnconnected=off
  ILE_sign : Outport  Port=3  VectorParamsAs1DForOutWhenUnconnected=off
  MPE1 : Outport  Port=4  VectorParamsAs1DForOutWhenUnconnected=off
  MPE1_sign : Outport  Port=5  VectorParamsAs1DForOutWhenUnconnected=off
  MPE2 : Outport  Port=6  VectorParamsAs1DForOutWhenUnconnected=off
  MPE2_sign : Outport  Port=7  VectorParamsAs1DForOutWhenUnconnected=off
  MPE3 : Outport  Port=8  VectorParamsAs1DForOutWhenUnconnected=off
  MPE3_sign : Outport  Port=9  VectorParamsAs1DForOutWhenUnconnected=off
  MPE4 : Outport  Port=10  VectorParamsAs1DForOutWhenUnconnected=off
  MPE4_sign : Outport  Port=11  VectorParamsAs1DForOutWhenUnconnected=off
  wires:
  Integrator1/1 -> Add1/2
  Add3/1 -> Product4/2, xf/1, Product3/2, ecgnoise1/1, Add1/1
  Manual Switch/1 -> Add3/1
  Random Gauss noise/1 -> Manual Switch/1
  Constant/1 -> Manual Switch/2
  Product1/1 -> Add2/1
  Gain3/1 -> Integrator3/1
  Add1/1 -> Product3/1, Gain2/1
  Product5/1 -> Gain3/1
  Gain2/1 -> Add2/2
  Add2/1 -> Integrator1/1
  Product3/1 -> Product5/2
  Constant1/1 -> Product5/1
  Integrator3/1 -> Sign3/1, MPE1/1, Product1/2
  ILE_system/2(sign) -> ILE_sign/1
  ILE_system/1(exp) -> ILE/1
  differential tracker1/1(diff_estimate) -> Add8/1, ILE_system/1(In)
  xf/1 -> Product4/1, Product2/1, Product2/2
  Product2/1 -> Product7/2, Add4/1, G/1
  Product4/1 -> Add4/2
  Add4/1 -> Gain1/1
  Gain1/1 -> Add6/2, S/1
  G/1 -> Product6/1
  Integrator2/1 -> Sign1/1, MPE2/1, Product7/1, Product6/2
  Product6/1 -> Add5/1
  S/1 -> Add5/2
  Product7/1 -> Add6/1
  Add6/1 -> Gain4/1
  Add5/1 -> Add7/1
  Gain4/1 -> Add7/2
  Add7/1 -> Gain5/1
  Gain5/1 -> Integrator2/1
  Sign1/1 -> MPE2_sign/1
  Product8/1 -> Add8/2
  Add8/1 -> MATLAB Function/1(u)
  MATLAB Function/1(y) -> Product9/1
  Product9/1 -> Gain6/1
  Gain6/1 -> Integrator4/1
  Integrator4/1 -> Sign2/1, MPE3/1, Product8/1
  Sign2/1 -> MPE3_sign/1
  Sign3/1 -> MPE1_sign/1
  Integrator5/1 -> Product10/1, MPE4/1, Sign4/1
  Sign4/1 -> MPE4_sign/1
  Add9/1 -> Product9/2, Product8/2, Product1/1, Add3/2, differential tracker1/1(signal)
  Constant2/1 -> Add9/2
  differential tracker2/1(diff_estimate) -> Subsystem/2(y)
  Constant3/1 -> Subsystem/3(alpha)
  Constant4/1 -> Subsystem/4(beta)
  Subsystem/1(Phi21) -> Product11/2, Product10/2
  Product10/1 -> Add10/1
  Subsystem/2(Y2) -> Add10/2
  Add10/1 -> Product11/1
  Product11/1 -> Gain7/1
  Gain7/1 -> Integrator5/1
  x/1 -> Transfer Fcn/1, Out1/1
  Transfer Fcn/1 -> differential tracker2/1(signal), Subsystem/1(x), Add9/1

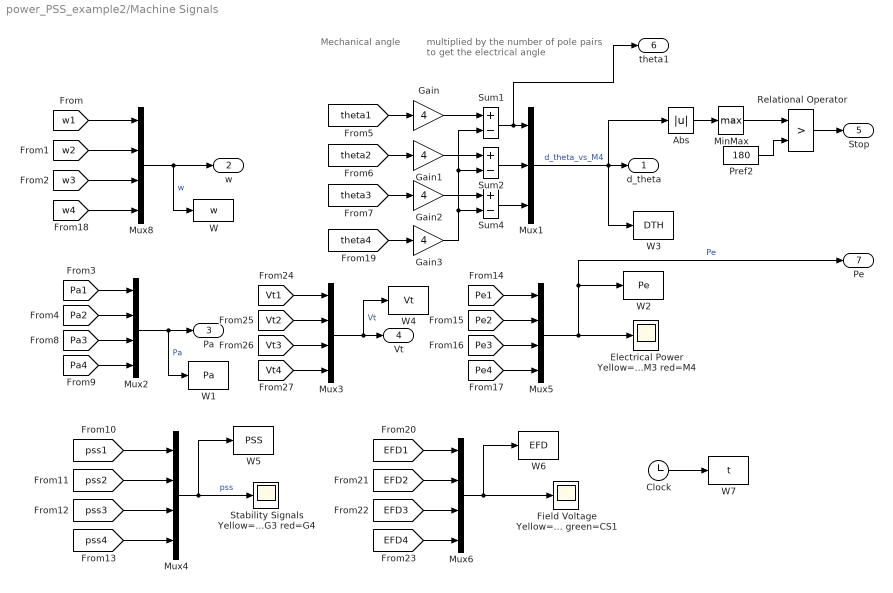
== system power_PSS_example2/Machine Signals ==
  note: Mechanical angle
  note: multiplied by the number of pole pairs
      | to get the electrical angle
  Abs : Abs
  Clock : Clock
  "Electrical Power Yellow=M1 mag=M2 cyan=M3 red=M4 " : Scope
  Field Voltage Yellow=G1 mag=G2 cyan=G3 red=G4 green=CS1 : Scope
  Gain{,1..3} (4 alike) : Gain  Gain=4
  MinMax : MinMax  Function=max  InputSameDT=on  SaturateOnIntegerOverflow=on
  Mux1 : Mux  Inputs=3
  Mux{2..6,8} (6 alike) : Mux
  Pref2 : Constant  Value=180
  Relational Operator : RelationalOperator  Operator=>
  "Stability Signals Yellow=G1 mag=G2 cyan=G3 red=G4 " : Scope
  Sum1 : Sum  Inputs=+-  InputSameDT=on  SaturateOnIntegerOverflow=on  OutDataTypeStr=Inherit: Same as first input
  Sum2 : Sum  Inputs=+-  InputSameDT=on  SaturateOnIntegerOverflow=on  OutDataTypeStr=Inherit: Same as first input
  Sum4 : Sum  Inputs=+-  InputSameDT=on  SaturateOnIntegerOverflow=on  OutDataTypeStr=Inherit: Same as first input
  W : ToWorkspace  VariableName=w  SampleTime=1/60
  W1 : ToWorkspace  VariableName=Pa  SampleTime=1/60
  W2 : ToWorkspace  VariableName=Pe  SampleTime=1/60
  W3 : ToWorkspace  VariableName=DTH  SampleTime=1/60
  W4 : ToWorkspace  VariableName=Vt  SampleTime=1/60
  W5 : ToWorkspace  VariableName=PSS  SampleTime=1/60
  W6 : ToWorkspace  VariableName=EFD  SampleTime=1/60
  W7 : ToWorkspace  VariableName=t  SampleTime=1/60
  d_theta : Outport  VectorParamsAs1DForOutWhenUnconnected=off
  w : Outport  Port=2  VectorParamsAs1DForOutWhenUnconnected=off
  Pa : Outport  Port=3  VectorParamsAs1DForOutWhenUnconnected=off
  Vt : Outport  Port=4  VectorParamsAs1DForOutWhenUnconnected=off
  Stop : Outport  Port=5  VectorParamsAs1DForOutWhenUnconnected=off
  theta1 : Outport  Port=6  VectorParamsAs1DForOutWhenUnconnected=off
  Pe : Outport  Port=7  VectorParamsAs1DForOutWhenUnconnected=off
  wires:
  Mux1/1 -> d_theta/1, Abs/1, W3/1  "d_theta_vs_M4"
  Abs/1 -> MinMax/1
  Pref2/1 -> Relational Operator/2
  MinMax/1 -> Relational Operator/1
  [Pa1] -> Mux2/1
  Mux4/1 -> "Stability Signals Yellow=G1 mag=G2 cyan=G3 red=G4 "/1, W5/1  "pss"
  [pss1] -> Mux4/1
  [pss2] -> Mux4/2
  [pss4] -> Mux4/4
  [pss3] -> Mux4/3
  [EFD1] -> Mux6/1
  [EFD2] -> Mux6/2
  [EFD4] -> Mux6/4
  [EFD3] -> Mux6/3
  Mux6/1 -> Field Voltage Yellow=G1 mag=G2 cyan=G3 red=G4 green=CS1/1, W6/1
  Mux8/1 -> w/1, W/1  "w"
  Relational Operator/1 -> Stop/1
  Mux2/1 -> Pa/1, W1/1  "Pa"
  [theta1] -> Gain/1
  Sum1/1 -> theta1/1, Mux1/1
  [theta2] -> Gain1/1
  [theta3] -> Gain2/1
  [theta4] -> Gain3/1
  Sum2/1 -> Mux1/2
  Sum4/1 -> Mux1/3
  [Pa2] -> Mux2/2
  [Pa3] -> Mux2/3
  [Pa4] -> Mux2/4
  [Vt1] -> Mux3/1
  [Vt2] -> Mux3/2
  [Vt3] -> Mux3/3
  [Vt4] -> Mux3/4
  Mux3/1 -> Vt/1, W4/1  "Vt"
  [Pe1] -> Mux5/1
  [Pe2] -> Mux5/2
  [Pe3] -> Mux5/3
  [Pe4] -> Mux5/4
  Mux5/1 -> "Electrical Power Yellow=M1 mag=M2 cyan=M3 red=M4 "/1, Pe/1, W2/1  "Pe"
  [w1] -> Mux8/1
  [w2] -> Mux8/2
  [w3] -> Mux8/3
  [w4] -> Mux8/4
  Clock/1 -> W7/1
  Gain/1 -> Sum1/1
  Gain1/1 -> Sum2/1
  Gain2/1 -> Sum4/1
  Gain3/1 -> Sum4/2, Sum2/2, Sum1/2

== system power_PSS_example2/SubSystem ==

== system power_PSS_example2/SubSystem3 ==

== system power_PSS_example2/SubSystem4 ==

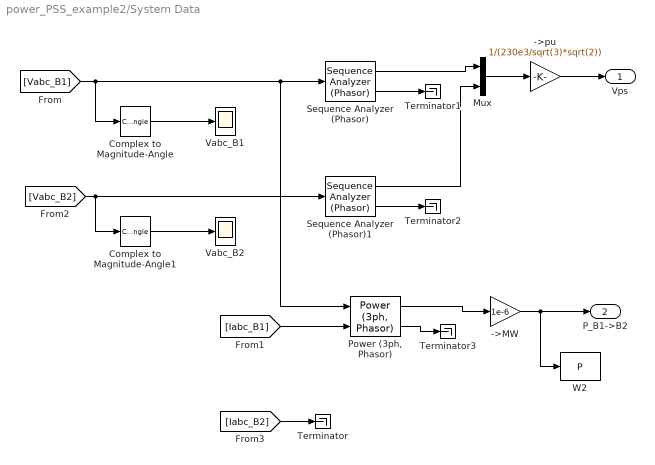
== system power_PSS_example2/System Data ==
  ->MW : Gain  Gain=1e-6  SaturateOnIntegerOverflow=on  OutDataTypeStr=Inherit: Same as input  ParamDataTypeStr=Inherit: Same as input
  ->pu : Gain  Gain=1/(230e3/sqrt(3)*sqrt(2))  SaturateOnIntegerOverflow=on  OutDataTypeStr=Inherit: Same as input  ParamDataTypeStr=Inherit: Same as input
  Complex to Magnitude-Angle : ComplexToMagnitudeAngle  Output=Magnitude
  Complex to Magnitude-Angle1 : ComplexToMagnitudeAngle  Output=Magnitude
  Mux : Mux  Inputs=2
  "Power (3ph, Phasor)" : spsPower3phPhasorLib/Power (3ph, Phasor)
      settings: SourceProductBaseCode=PS
  Sequence Analyzer (Phasor) : spsSequenceAnalyzerPhasorLib/Sequence Analyzer (Phasor)  seq=Positive
      settings: SourceProductBaseCode=PS
  Sequence Analyzer (Phasor)1 : spsSequenceAnalyzerPhasorLib/Sequence Analyzer (Phasor)  seq=Positive
      settings: SourceProductBaseCode=PS
  Terminator{,1..3} (4 alike) : Terminator
  Vabc_B1 : Scope
  Vabc_B2 : Scope
  W2 : ToWorkspace  VariableName=P  SampleTime=1/60
  Vps : Outport  VectorParamsAs1DForOutWhenUnconnected=off
  P_B1->B2 : Outport  Port=2  VectorParamsAs1DForOutWhenUnconnected=off
  wires:
  [Vabc_B1] -> Sequence Analyzer (Phasor)/1, "Power (3ph, Phasor)"/1, Complex to Magnitude-Angle/1
  [Vabc_B2] -> Sequence Analyzer (Phasor)1/1, Complex to Magnitude-Angle1/1
  [Iabc_B2] -> Terminator/1
  Sequence Analyzer (Phasor)/2 -> Terminator1/1
  Sequence Analyzer (Phasor)1/2 -> Terminator2/1
  Sequence Analyzer (Phasor)1/1 -> Mux/2
  [Iabc_B1] -> "Power (3ph, Phasor)"/2
  Sequence Analyzer (Phasor)/1 -> Mux/1
  Mux/1 -> ->pu/1
  ->MW/1 -> P_B1->B2/1, W2/1
  Complex to Magnitude-Angle/1 -> Vabc_B1/1
  Complex to Magnitude-Angle1/1 -> Vabc_B2/1
  "Power (3ph, Phasor)"/1 -> ->MW/1
  "Power (3ph, Phasor)"/2 -> Terminator3/1
  ->pu/1 -> Vps/1

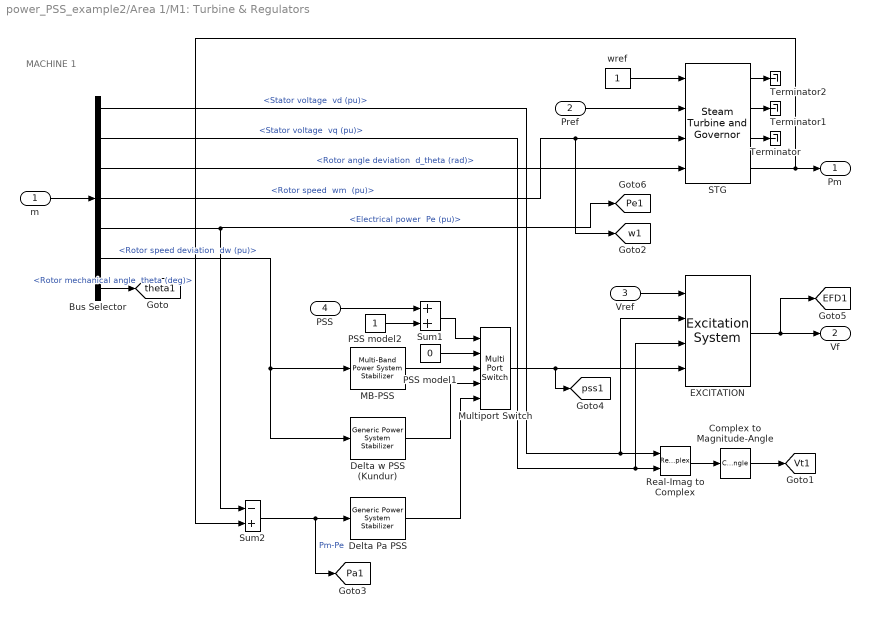
== system power_PSS_example2/Area 1/M1: Turbine & Regulators ==
  note: MACHINE 1
  m : Inport
  Pref : Inport  Port=2
  Vref : Inport  Port=3
  PSS : Inport  Port=4
  Bus Selector : BusSelector  OutputSignals="dq0 components.Stator voltage  vd (pu),dq0 components.Stator voltage  vq (pu),Mechanical.Rotor angle deviation  d_theta (rad),Mechanical.Rotor speed  wm  (pu),Mechanical.Electrical power  Pe (pu),Mechanical.Rotor speed deviation  dw (pu),Mechanical.Rotor mechanical angle  theta (deg)"
  Complex to Magnitude-Angle : ComplexToMagnitudeAngle  Output=Magnitude
  "Delta Pa PSS " : spsGenericPowerSystemStabilizerLib/Generic Power System Stabilizer  Tsensor=15e-3  K=2.5*1.25  Twashout=1  Tleadlag1=[60e-3 1]  Tleadlag2=[0 0]  VSlimits=[-0.15 0.15]  Vinit=0  Plot_On=off  MagdB_On=off  FreqRange=logspace(-2,2,500)
      settings: SourceProductBaseCode=PS
  "Delta w PSS (Kundur) " : spsGenericPowerSystemStabilizerLib/Generic Power System Stabilizer  Tsensor=15e-3  K=30  Twashout=10  Tleadlag1=[50e-3 20e-3]  Tleadlag2=[3 5.4]  VSlimits=[-0.15 0.15]  Vinit=0  Plot_On=off  MagdB_On=off  FreqRange=logspace(-2,2,500)
      settings: SourceProductBaseCode=PS
  EXCITATION : spsExcitationSystemLib/Excitation System  tr=20e-3  reg=[ 200, 0.001 ]  exc=[ 1, 0 ]  tgr=[ 0, 0 ]  damp=[ 0, 0 ]  sat=[ 0, 0 ]  lim=[ 0 , 12.3, 0 ]  v0=[1,1.83395]
      settings: SourceProductBaseCode=PS
  "MB-PSS " : spsMultiBandPowerSystemStabilizerLib/Multi-Band Power System Stabilizer  OperationMode=Simplified settings  Kg=1.0  GL=[0.2 30]  GI=[1.25 40]  GH=[12.0 160]  GLd=[66 66 9.4]  TcLF=[1.667 2 0 0 0 0 2 2.4 0 0 0 0 1 1]  GId=[66 66 47.6]  TcIF=[1 1 0.25 0.3 0 0 1 1 0.3 0.36 0 0 0 0]  GHd=[66 66 233]  TcHF="[0.01 0.012 0 0 0 0  0.012 0.0144 0 0 0 0 1 1]"  LIM=[.075 .15 .15 .15]  Plot_On=off  MagdB_On=off  FreqRange=logspace(-2,2,500)
      settings: SourceProductBaseCode=PS
  Multiport Switch : MultiPortSwitch  Inputs=4  SaturateOnIntegerOverflow=off
  PSS model1 : Constant  Value=0
  PSS model2 : Constant
  Real-Imag to Complex : RealImagToComplex
  STG : spsSteamTurbineandGovernorLib/Steam Turbine and Governor  gentype=Tandem-compound (single mass)  reg1="[ 1  0.05    0 ]"  reg2="[ 0.001  0.15 ]"  reg3="[ -0.1  0.1  0  4.496 ]"  N=3600  turb1="[ 0  10   3.3   0.5   ]"  turb2="[   0   0.36    0.36   0.28   ]"  HA="[ 0.046  1.430  1.465   0.192 ]"  KA="[ 90.44  53.88  64.59   62.94  ]"  DA="[ 0.0115  0.3575  0.3663   0.0137  ]"  ini1=0.7778  ini2=[0.779316,-31.4247]
      settings: SourceProductBaseCode=PS
  Sum1 : Sum  InputSameDT=on  SaturateOnIntegerOverflow=on  OutDataTypeStr=Inherit: Same as first input
  Sum2 : Sum  Inputs=-+  InputSameDT=on  SaturateOnIntegerOverflow=on  OutDataTypeStr=Inherit: Same as first input
  Terminator : Terminator
  Terminator1 : Terminator
  Terminator2 : Terminator
  wref : Constant
  Pm : Outport  InitialOutput=0  VectorParamsAs1DForOutWhenUnconnected=off
  Vf : Outport  Port=2  InitialOutput=0  VectorParamsAs1DForOutWhenUnconnected=off
  tag scope: EFD1=global, Pa1=global, Pe1=global, Vt1=global, pss1=global, theta1=global, w1=global
  wires:
  Bus Selector/1 -> Real-Imag to Complex/1, EXCITATION/2  "<Stator voltage  vd (pu)>"
  Bus Selector/2 -> Real-Imag to Complex/2, EXCITATION/3  "<Stator voltage  vq (pu)>"
  wref/1 -> STG/1
  Pref/1 -> STG/2
  m/1 -> Bus Selector/1
  Vref/1 -> EXCITATION/1
  Real-Imag to Complex/1 -> Complex to Magnitude-Angle/1
  EXCITATION/1 -> Vf/1, [EFD1]
  Complex to Magnitude-Angle/1 -> [Vt1]
  Bus Selector/7 -> [theta1]  "<Rotor mechanical angle  theta (deg)>"
  Multiport Switch/1 -> EXCITATION/4, [pss1]
  PSS model1/1 -> Multiport Switch/2
  "MB-PSS "/1 -> Multiport Switch/3
  "Delta w PSS (Kundur) "/1 -> Multiport Switch/4
  "Delta Pa PSS "/1 -> Multiport Switch/5
  PSS model2/1 -> Sum1/2
  Sum1/1 -> Multiport Switch/1
  PSS/1 -> Sum1/1
  Bus Selector/4 -> [w1], STG/3  "<Rotor speed  wm  (pu)>"
  Bus Selector/5 -> [Pe1], Sum2/1  "<Electrical power  Pe (pu)>"
  Bus Selector/6 -> "Delta w PSS (Kundur) "/1, "MB-PSS "/1  "<Rotor speed deviation  dw (pu)>"
  Sum2/1 -> [Pa1], "Delta Pa PSS "/1  "Pm-Pe"
  STG/3 -> Terminator/1
  STG/4 -> Pm/1, Sum2/2
  STG/2 -> Terminator1/1
  STG/1 -> Terminator2/1
  Bus Selector/3 -> STG/4  "<Rotor angle deviation  d_theta (rad)>"

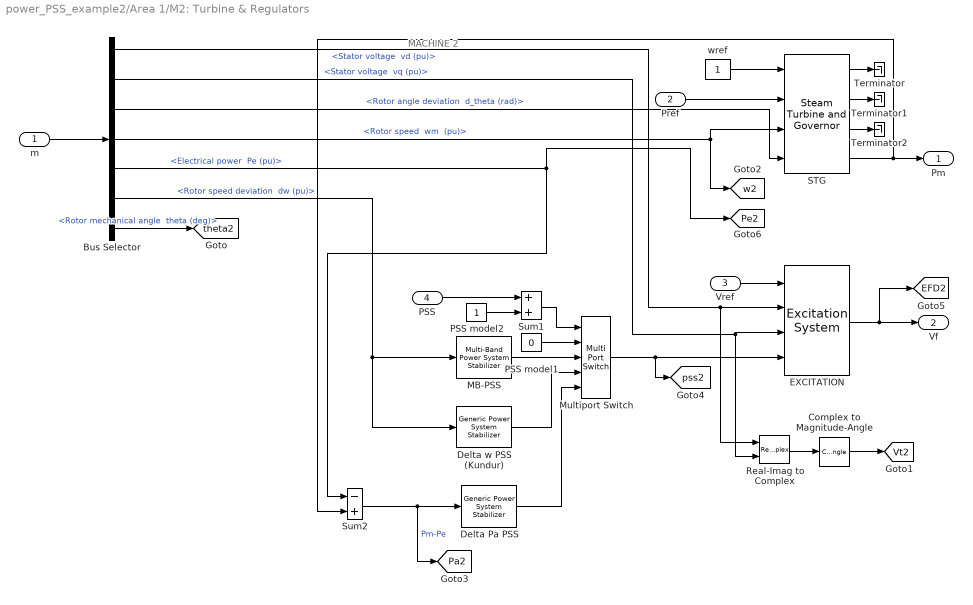
== system power_PSS_example2/Area 1/M2: Turbine & Regulators ==
  note: MACHINE 2
  m : Inport
  Pref : Inport  Port=2
  Vref : Inport  Port=3
  PSS : Inport  Port=4
  Bus Selector : BusSelector  OutputSignals="dq0 components.Stator voltage  vd (pu),dq0 components.Stator voltage  vq (pu),Mechanical.Rotor angle deviation  d_theta (rad),Mechanical.Rotor speed  wm  (pu),Mechanical.Electrical power  Pe (pu),Mechanical.Rotor speed deviation  dw (pu),Mechanical.Rotor mechanical angle  theta (deg)"
  Complex to Magnitude-Angle : ComplexToMagnitudeAngle  Output=Magnitude
  "Delta Pa PSS " : spsGenericPowerSystemStabilizerLib/Generic Power System Stabilizer  Tsensor=15e-3  K=2.5*1.25  Twashout=1  Tleadlag1=[60e-3 1]  Tleadlag2=[0 0]  VSlimits=[-0.15 0.15]  Vinit=0  Plot_On=off  MagdB_On=on  FreqRange=logspace(-2,2,500)
      settings: SourceProductBaseCode=PS
  "Delta w PSS (Kundur) " : spsGenericPowerSystemStabilizerLib/Generic Power System Stabilizer  Tsensor=15e-3  K=30  Twashout=10  Tleadlag1=[50e-3 20e-3]  Tleadlag2=[3 5.4]  VSlimits=[-0.15 0.15]  Vinit=0  Plot_On=off  MagdB_On=on  FreqRange=logspace(-2,2,500)
      settings: SourceProductBaseCode=PS
  EXCITATION : spsExcitationSystemLib/Excitation System  tr=20e-3  reg=[ 200, 0.001 ]  exc=[ 1, 0 ]  tgr=[ 0, 0 ]  damp=[ 0, 0 ]  sat=[ 0, 0 ]  lim=[ 0 , 12.3, 0 ]  v0=[1,1.86756]
      settings: SourceProductBaseCode=PS
  "MB-PSS " : spsMultiBandPowerSystemStabilizerLib/Multi-Band Power System Stabilizer  OperationMode=Simplified settings  Kg=1.0  GL=[0.2 30]  GI=[1.25 40]  GH=[12.0 160]  GLd=[66 66 9.4]  TcLF=[1.667 2 0 0 0 0 2 2.4 0 0 0 0 1 1]  GId=[66 66 47.6]  TcIF=[1 1 0.25 0.3 0 0 1 1 0.3 0.36 0 0 0 0]  GHd=[66 66 233]  TcHF="[0.01 0.012 0 0 0 0  0.012 0.0144 0 0 0 0 1 1]"  LIM=[.075 .15 .15 .15]  Plot_On=off  MagdB_On=off  FreqRange=logspace(-2,2,500)
      settings: SourceProductBaseCode=PS
  Multiport Switch : MultiPortSwitch  Inputs=4  SaturateOnIntegerOverflow=off
  PSS model1 : Constant  Value=0
  PSS model2 : Constant
  Real-Imag to Complex : RealImagToComplex
  STG : spsSteamTurbineandGovernorLib/Steam Turbine and Governor  gentype=Tandem-compound (single mass)  reg1="[ 1  0.05    0 ]"  reg2="[ 0.001  0.15 ]"  reg3="[ -0.1  0.1  0  4.496 ]"  N=3600  turb1="[ 0  10   3.3   0.5   ]"  turb2="[   0   0.36    0.36   0.28   ]"  HA="[ 0.046  1.430  1.465   0.192 ]"  KA="[ 90.44  53.88  64.59   62.94  ]"  DA="[ 0.0115  0.3575  0.3663   0.0137  ]"  ini1=0.7777  ini2=[0.779243,-42.8075]
      settings: SourceProductBaseCode=PS
  Sum1 : Sum  InputSameDT=on  SaturateOnIntegerOverflow=on  OutDataTypeStr=Inherit: Same as first input
  Sum2 : Sum  Inputs=-+  InputSameDT=on  SaturateOnIntegerOverflow=on  OutDataTypeStr=Inherit: Same as first input
  Terminator : Terminator
  Terminator1 : Terminator
  Terminator2 : Terminator
  wref : Constant
  Pm : Outport  InitialOutput=0  VectorParamsAs1DForOutWhenUnconnected=off
  Vf : Outport  Port=2  InitialOutput=0  VectorParamsAs1DForOutWhenUnconnected=off
  tag scope: EFD2=global, Pa2=global, Pe2=global, Vt2=global, pss2=global, theta2=global, w2=global
  wires:
  Sum2/1 -> [Pa2], "Delta Pa PSS "/1  "Pm-Pe"
  Bus Selector/6 -> "MB-PSS "/1, "Delta w PSS (Kundur) "/1  "<Rotor speed deviation  dw (pu)>"
  Bus Selector/5 -> [Pe2], Sum2/1  "<Electrical power  Pe (pu)>"
  Bus Selector/4 -> STG/3, [w2]  "<Rotor speed  wm  (pu)>"
  PSS/1 -> Sum1/1
  Sum1/1 -> Multiport Switch/1
  PSS model2/1 -> Sum1/2
  "Delta Pa PSS "/1 -> Multiport Switch/5
  "Delta w PSS (Kundur) "/1 -> Multiport Switch/4
  "MB-PSS "/1 -> Multiport Switch/3
  PSS model1/1 -> Multiport Switch/2
  Multiport Switch/1 -> [pss2], EXCITATION/4
  Bus Selector/7 -> [theta2]  "<Rotor mechanical angle  theta (deg)>"
  Complex to Magnitude-Angle/1 -> [Vt2]
  EXCITATION/1 -> [EFD2], Vf/1
  Real-Imag to Complex/1 -> Complex to Magnitude-Angle/1
  Vref/1 -> EXCITATION/1
  Pref/1 -> STG/2
  wref/1 -> STG/1
  Bus Selector/2 -> Real-Imag to Complex/2, EXCITATION/3  "<Stator voltage  vq (pu)>"
  Bus Selector/1 -> Real-Imag to Complex/1, EXCITATION/2  "<Stator voltage  vd (pu)>"
  STG/1 -> Terminator/1
  STG/2 -> Terminator1/1
  STG/3 -> Terminator2/1
  STG/4 -> Pm/1, Sum2/2
  Bus Selector/3 -> STG/4  "<Rotor angle deviation  d_theta (rad)>"
  m/1 -> Bus Selector/1

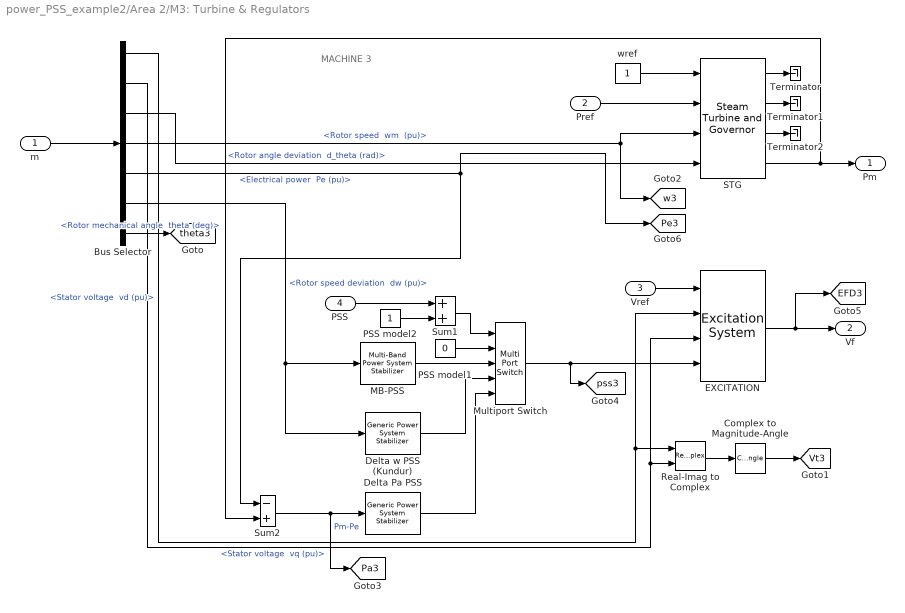
== system power_PSS_example2/Area 2/M3: Turbine & Regulators ==
  note: MACHINE 3
  m : Inport
  Pref : Inport  Port=2
  Vref : Inport  Port=3
  PSS : Inport  Port=4
  Bus Selector : BusSelector  OutputSignals="dq0 components.Stator voltage  vd (pu),dq0 components.Stator voltage  vq (pu),Mechanical.Rotor angle deviation  d_theta (rad),Mechanical.Rotor speed  wm  (pu),Mechanical.Electrical power  Pe (pu),Mechanical.Rotor speed deviation  dw (pu),Mechanical.Rotor mechanical angle  theta (deg)"
  Complex to Magnitude-Angle : ComplexToMagnitudeAngle  Output=Magnitude
  "Delta Pa PSS " : spsGenericPowerSystemStabilizerLib/Generic Power System Stabilizer  Tsensor=15e-3  K=2.5*1.25  Twashout=1  Tleadlag1=[60e-3 1]  Tleadlag2=[0 0]  VSlimits=[-0.15 0.15]  Vinit=0  Plot_On=off  MagdB_On=on  FreqRange=logspace(-2,2,500)
      settings: SourceProductBaseCode=PS
  "Delta w PSS (Kundur) " : spsGenericPowerSystemStabilizerLib/Generic Power System Stabilizer  Tsensor=15e-3  K=30  Twashout=10  Tleadlag1=[50e-3 20e-3]  Tleadlag2=[3 5.4]  VSlimits=[-0.15 0.15]  Vinit=0  Plot_On=off  MagdB_On=on  FreqRange=logspace(-2,2,500)
      settings: SourceProductBaseCode=PS
  EXCITATION : spsExcitationSystemLib/Excitation System  tr=20e-3  reg=[ 200, 0.001 ]  exc=[ 1, 0 ]  tgr=[ 0, 0 ]  damp=[ 0, 0 ]  sat=[ 0, 0 ]  lim=[ 0 , 12.3, 0 ]  v0=[1,1.85092]
      settings: SourceProductBaseCode=PS
  "MB-PSS " : spsMultiBandPowerSystemStabilizerLib/Multi-Band Power System Stabilizer  OperationMode=Simplified settings  Kg=1.0  GL=[0.2 30]  GI=[1.25 40]  GH=[12.0 160]  GLd=[66 66 9.4]  TcLF=[1.667 2 0 0 0 0 2 2.4 0 0 0 0 1 1]  GId=[66 66 47.6]  TcIF=[1 1 0.25 0.3 0 0 1 1 0.3 0.36 0 0 0 0]  GHd=[66 66 233]  TcHF="[0.01 0.012 0 0 0 0  0.012 0.0144 0 0 0 0 1 1]"  LIM=[.075 .15 .15 .15]  Plot_On=off  MagdB_On=off  FreqRange=logspace(-2,2,500)
      settings: SourceProductBaseCode=PS
  Multiport Switch : MultiPortSwitch  Inputs=4  SaturateOnIntegerOverflow=off
  PSS model1 : Constant  Value=0
  PSS model2 : Constant
  Real-Imag to Complex : RealImagToComplex
  STG : spsSteamTurbineandGovernorLib/Steam Turbine and Governor  gentype=Tandem-compound (single mass)  reg1="[ 1  0.05    0 ]"  reg2="[ 0.001  0.15 ]"  reg3="[ -0.1  0.1  0  4.496 ]"  N=3600  turb1="[ 0  10   3.3   0.5   ]"  turb2="[   0   0.36    0.36   0.28   ]"  HA="[ 0.046  1.430  1.465   0.192 ]"  KA="[ 90.44  53.88  64.59   62.94  ]"  DA="[ 0.0115  0.3575  0.3663   0.0137  ]"  ini1=0.798889  ini2=[0.800505,-56.3243]
      settings: SourceProductBaseCode=PS
  Sum1 : Sum  InputSameDT=on  SaturateOnIntegerOverflow=on  OutDataTypeStr=Inherit: Same as first input
  Sum2 : Sum  Inputs=-+  InputSameDT=on  SaturateOnIntegerOverflow=on  OutDataTypeStr=Inherit: Same as first input
  Terminator : Terminator
  Terminator1 : Terminator
  Terminator2 : Terminator
  wref : Constant
  Pm : Outport  InitialOutput=0  VectorParamsAs1DForOutWhenUnconnected=off
  Vf : Outport  Port=2  InitialOutput=0  VectorParamsAs1DForOutWhenUnconnected=off
  tag scope: EFD3=global, Pa3=global, Pe3=global, Vt3=global, pss3=global, theta3=global, w3=global
  wires:
  Sum2/1 -> [Pa3], "Delta Pa PSS "/1  "Pm-Pe"
  Bus Selector/6 -> "MB-PSS "/1, "Delta w PSS (Kundur) "/1  "<Rotor speed deviation  dw (pu)>"
  Bus Selector/5 -> [Pe3], Sum2/1  "<Electrical power  Pe (pu)>"
  Bus Selector/4 -> STG/3, [w3]  "<Rotor speed  wm  (pu)>"
  PSS/1 -> Sum1/1
  Sum1/1 -> Multiport Switch/1
  PSS model2/1 -> Sum1/2
  "Delta Pa PSS "/1 -> Multiport Switch/5
  "Delta w PSS (Kundur) "/1 -> Multiport Switch/4
  "MB-PSS "/1 -> Multiport Switch/3
  PSS model1/1 -> Multiport Switch/2
  Multiport Switch/1 -> [pss3], EXCITATION/4
  Bus Selector/7 -> [theta3]  "<Rotor mechanical angle  theta (deg)>"
  Complex to Magnitude-Angle/1 -> [Vt3]
  EXCITATION/1 -> [EFD3], Vf/1
  Real-Imag to Complex/1 -> Complex to Magnitude-Angle/1
  Vref/1 -> EXCITATION/1
  Pref/1 -> STG/2
  wref/1 -> STG/1
  Bus Selector/2 -> EXCITATION/3, Real-Imag to Complex/2  "<Stator voltage  vq (pu)>"
  Bus Selector/1 -> EXCITATION/2, Real-Imag to Complex/1  "<Stator voltage  vd (pu)>"
  Bus Selector/3 -> STG/4  "<Rotor angle deviation  d_theta (rad)>"
  STG/1 -> Terminator/1
  STG/2 -> Terminator1/1
  STG/3 -> Terminator2/1
  STG/4 -> Pm/1, Sum2/2
  m/1 -> Bus Selector/1
